simulink model "SIL"  (R2023a)
settings: Solver=FixedStepDiscrete  StartTime=0.0  StopTime=10.0  FixedStep=0.01  RelTol=1e-3
libraries: pil_lib x1
settings Model: Creator=eslam  LastModifiedBy=eslam
settings OptimizationCC: DefaultParameterBehavior=Inlined  UseDivisionForNetSlopeComputation=on  GainParamInheritBuiltInType=on  UseFloatMulNetSlope=on  InlineInvariantSignals=on  PassReuseOutputArgsAs=Individual arguments  ZeroExternalMemoryAtStartup=off  ZeroInternalMemoryAtStartup=off  NoFixptDivByZeroProtection=on  EfficientFloat2IntCast=on  LifeSpan=1  OptimizeBlockOrder=speed  DifferentSizesBufferReuse=on  EfficientTunableParamExpr=on
settings DebuggingCC: ParameterTunabilityLossMsg=error
settings HardwareCC: ProdLongLongMode=on
settings SFSimCC: MATLABDynamicMemAlloc=off
settings RTWCC: Description=Embedded Coder  SystemTargetFile=ert.tlc  TemplateMakefile=ert_default_tmf
settings CodeAppCC: ForceParamTrailComments=on  IgnoreCustomStorageClasses=off  OperatorAnnotations=on  SimulinkDataObjDesc=on  SFDataObjDesc=on  CustomSymbolStrGlobalVar=rt$N$M  CustomSymbolStrType=$N$M  CustomSymbolStrFcn=$N$M$F  CustomSymbolStrMacro=$N$M  InsertBlockDesc=on
settings ERTTargetCC: TargetLangStandard=C99 (ISO)  GenerateSampleERTMain=on  IncludeMdlTerminateFcn=off  CombineSignalStateStructs=on  SuppressErrorStatus=on  SupportAbsoluteTime=off  SupportComplex=off  InlinedParameterPlacement=NonHierarchical  ERTCustomFileTemplate=example_file_process.tlc  ERTFilePackagingFormat=CompactWithDataFile

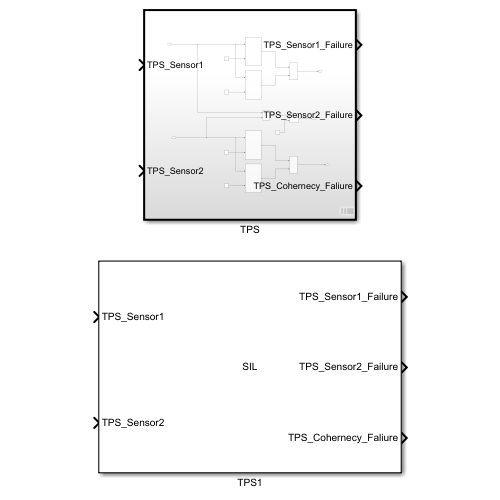
[thumbnail: Simulink's stored preview of the top-level diagram]
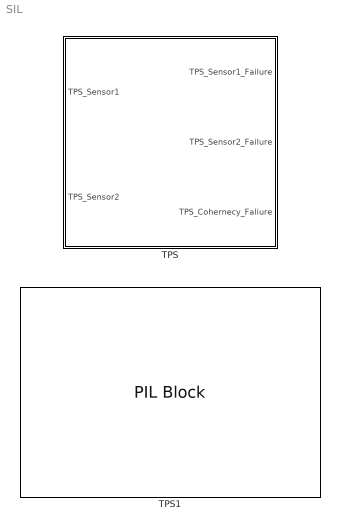
== system SIL ==
  TPS : Subsystem  TreatAsAtomicUnit=on
  TPS1 : pil_lib/PIL Block  Tag=__SL_testing_harness_stub_  SimulationMode=SIL  IsTopModelPIL=off  CodeDir=C:\Users\eslam\Desktop\New folder\TPS_ert_rtw  AnchorDir=C:\Users\eslam\Desktop\New folder\xrel  ConfigName=Software-in-the-Loop (SIL)  XRelSourceFile=C:\Users\eslam\Desktop\New folder\TPS_ert_rtw\TPS.c  XrelIsTopModelCode=on  XrelIsReusable=off  XrelDWorkNames={}  XrelDWorkTypes={}  XrelModelArgVals={}  XrelOrderedParamNames={}  XILSFunction=TPS_R2023a_sil

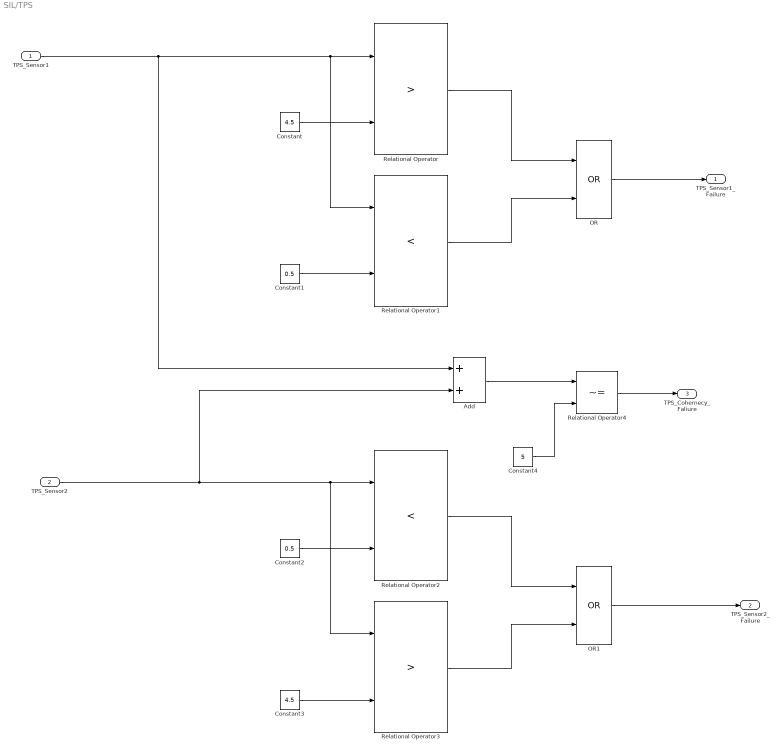
== system SIL/TPS ==
  TPS_Sensor1 : Inport  OutDataTypeStr=single
  TPS_Sensor2 : Inport  Port=2  OutDataTypeStr=single
  Add : Sum
  Constant : Constant  Value=4.5
  Constant1 : Constant  Value=0.5
  Constant2 : Constant  Value=0.5
  Constant3 : Constant  Value=4.5
  Constant4 : Constant  Value=5
  OR : Logic  Operator=OR  AllPortsSameDT=off  OutDataTypeStr=boolean
  OR1 : Logic  Operator=OR  AllPortsSameDT=off  OutDataTypeStr=boolean
  Relational Operator : RelationalOperator  Operator=>  OutDataTypeStr=boolean  RndMeth=Simplest  InputSameDT=off
  Relational Operator1 : RelationalOperator  Operator=<  OutDataTypeStr=boolean  RndMeth=Simplest  InputSameDT=off
  Relational Operator2 : RelationalOperator  Operator=<  OutDataTypeStr=boolean  RndMeth=Simplest  InputSameDT=off
  Relational Operator3 : RelationalOperator  Operator=>  OutDataTypeStr=boolean  RndMeth=Simplest  InputSameDT=off
  Relational Operator4 : RelationalOperator  Operator=~=  OutDataTypeStr=boolean  RndMeth=Simplest  InputSameDT=off
  TPS_Sensor1_Failure : Outport  OutDataTypeStr=boolean
  TPS_Sensor2_Failure : Outport  Port=2  OutDataTypeStr=boolean
  TPS_Cohernecy_Faliure : Outport  Port=3  OutDataTypeStr=boolean
  wires:
  Constant/1 -> Relational Operator/2
  OR/1 -> TPS_Sensor1_Failure/1
  Relational Operator/1 -> OR/1
  Constant1/1 -> Relational Operator1/2
  Relational Operator1/1 -> OR/2
  TPS_Sensor1/1 -> Add/1, Relational Operator1/1, Relational Operator/1
  Constant3/1 -> Relational Operator3/2
  Constant2/1 -> Relational Operator2/2
  Relational Operator2/1 -> OR1/1
  TPS_Sensor2/1 -> Add/2, Relational Operator3/1, Relational Operator2/1
  Relational Operator3/1 -> OR1/2
  OR1/1 -> TPS_Sensor2_Failure/1
  Add/1 -> Relational Operator4/1
  Constant4/1 -> Relational Operator4/2
  Relational Operator4/1 -> TPS_Cohernecy_Faliure/1
